simulink library "Propulsion"  (R2024b)
settings: Solver=VariableStepAuto  StartTime=0.0  StopTime=10.0  RelTol=1e-3
undefined symbols (not defined in the file): alfaf_deg, nrho, nv, rho_reference_kgpm3, Tmax, V_reference_mps, xf_m, zf_m
settings Model: Creator=ada09  LastModifiedBy=ada09

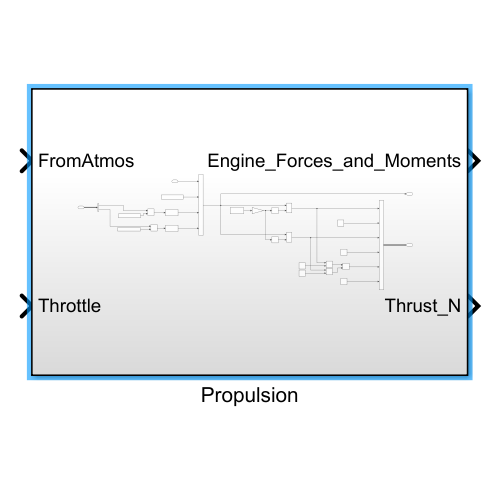
[thumbnail: Simulink's stored preview of the top-level diagram]
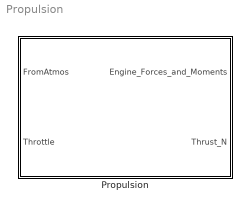
== system Propulsion ==
  Propulsion : Subsystem

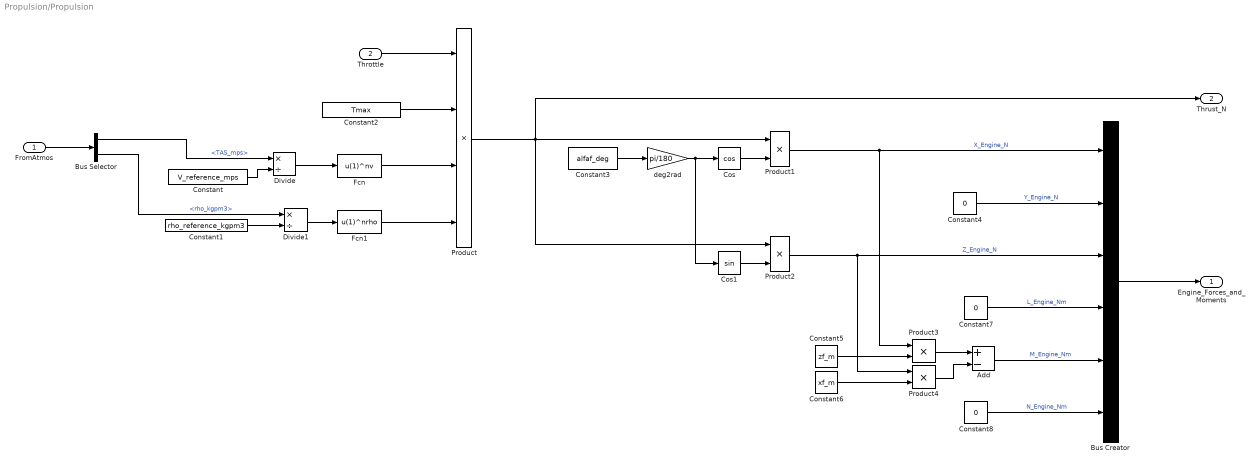
== system Propulsion/Propulsion ==
  FromAtmos : Inport
  Throttle : Inport  Port=2
  Add : Sum  Inputs=+-
  Bus Creator : BusCreator  Inputs=6
  Bus Selector : BusSelector  OutputSignals=TAS_mps,rho_kgpm3
  Constant : Constant  Value=V_reference_mps
  Constant1 : Constant  Value=rho_reference_kgpm3
  Constant2 : Constant  Value=Tmax
  Constant3 : Constant  Value=alfaf_deg
  Constant4 : Constant  Value=0
  Constant5 : Constant  Value=zf_m
  Constant6 : Constant  Value=xf_m
  Constant7 : Constant  Value=0
  Constant8 : Constant  Value=0
  Cos : Trigonometry  Operator=cos
  Cos1 : Trigonometry
  Divide : Product  Inputs=*/
  Divide1 : Product  Inputs=*/
  Fcn : Fcn  Expr=u(1)^nv
  Fcn1 : Fcn  Expr=u(1)^nrho
  Product : Product  Inputs=4
  Product{1..4} (4 alike) : Product
  deg2rad : Gain  Gain=pi/180
  Engine_Forces_and_Moments : Outport
  Thrust_N : Outport  Port=2
  wires:
  Constant5/1 -> Product3/2
  Constant6/1 -> Product4/2
  Cos1/1 -> Product2/2
  Constant7/1 -> Bus Creator/4  "L_Engine_Nm"
  Bus Creator/1 -> Engine_Forces_and_Moments/1
  Product4/1 -> Add/2
  Divide/1 -> Fcn/1
  Bus Selector/2 -> Divide1/1  "<rho_kgpm3>"
  deg2rad/1 -> Cos1/1, Cos/1
  Product2/1 -> Bus Creator/3, Product4/1  "Z_Engine_N"
  FromAtmos/1 -> Bus Selector/1
  Constant2/1 -> Product/2
  Product/1 -> Product2/1, Thrust_N/1, Product1/1
  Throttle/1 -> Product/1
  Bus Selector/1 -> Divide/1  "<TAS_mps>"
  Divide1/1 -> Fcn1/1
  Fcn1/1 -> Product/4
  Cos/1 -> Product1/2
  Constant3/1 -> deg2rad/1
  Fcn/1 -> Product/3
  Constant/1 -> Divide/2
  Product1/1 -> Bus Creator/1, Product3/1  "X_Engine_N"
  Constant1/1 -> Divide1/2
  Constant8/1 -> Bus Creator/6  "N_Engine_Nm"
  Constant4/1 -> Bus Creator/2  "Y_Engine_N"
  Add/1 -> Bus Creator/5  "M_Engine_Nm"
  Product3/1 -> Add/1
